simulink model "saturation_mdl"  (R2014a)
settings: Solver=ode45  StartTime=0.0  StopTime=10.0  RelTol=1e-3
values from neighbouring files (symbols this model uses):
  Kg_load_man = 150.5    [simulation.m]
  Kg_noload_man = 245.5    [simulation.m]
libraries: cstblocks x8
settings Model: Creator=daniw  LastModifiedBy=Nino
settings DebuggingCC: UnderspecifiedInitializationDetection=Classic

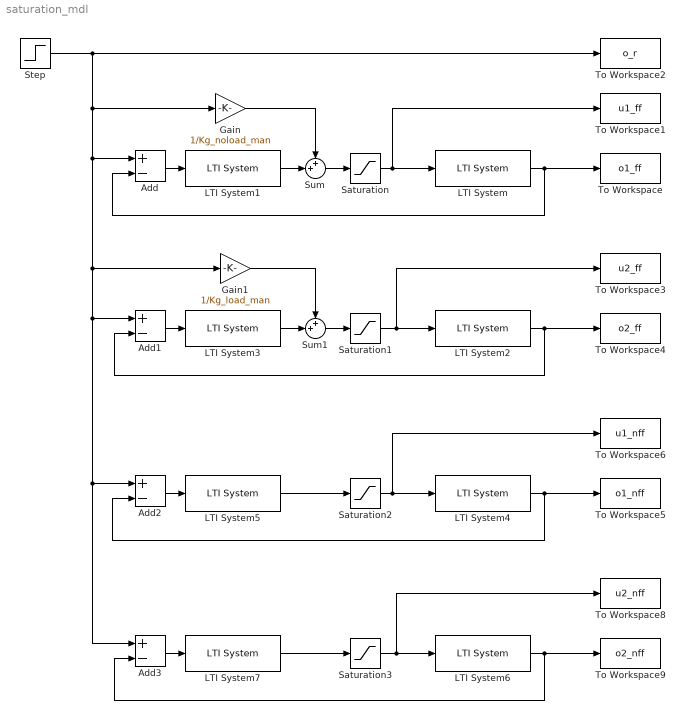
== system saturation_mdl ==
  Add{,1..3} (4 alike) : Sum  Inputs=+-
  Gain : Gain  Gain=1/Kg_noload_man
  Gain1 : Gain  Gain=1/Kg_load_man
  LTI System : cstblocks/LTI System  sys=G11_man  IC=[]
  LTI System{1,3,5,7} (4 alike) : cstblocks/LTI System  sys=C_PI  IC=[]
  LTI System2 : cstblocks/LTI System  sys=G12_man  IC=[]
  LTI System4 : cstblocks/LTI System  sys=G11_man  IC=[]
  LTI System6 : cstblocks/LTI System  sys=G12_man  IC=[]
  Saturation{,1..3} (4 alike) : Saturate  UpperLimit=24  LowerLimit=-24
  Step : Step  After=2500  SampleTime=0
  Sum : Sum  Inputs=++|
  Sum1 : Sum  Inputs=++|
  To Workspace : ToWorkspace  VariableName=o1_ff  SaveFormat=Structure With Time  SampleTime=-1
  To Workspace1 : ToWorkspace  VariableName=u1_ff  SaveFormat=Structure With Time  SampleTime=-1
  To Workspace2 : ToWorkspace  VariableName=o_r  SaveFormat=Structure With Time  SampleTime=-1
  To Workspace3 : ToWorkspace  VariableName=u2_ff  SaveFormat=Structure With Time  SampleTime=-1
  To Workspace4 : ToWorkspace  VariableName=o2_ff  SaveFormat=Structure With Time  SampleTime=-1
  To Workspace5 : ToWorkspace  VariableName=o1_nff  SaveFormat=Structure With Time  SampleTime=-1
  To Workspace6 : ToWorkspace  VariableName=u1_nff  SaveFormat=Structure With Time  SampleTime=-1
  To Workspace8 : ToWorkspace  VariableName=u2_nff  SaveFormat=Structure With Time  SampleTime=-1
  To Workspace9 : ToWorkspace  VariableName=o2_nff  SaveFormat=Structure With Time  SampleTime=-1
  wires:
  Add/1 -> LTI System1/1
  Saturation/1 -> To Workspace1/1, LTI System/1
  LTI System/1 -> To Workspace/1, Add/2
  Add1/1 -> LTI System3/1
  Saturation1/1 -> To Workspace3/1, LTI System2/1
  LTI System2/1 -> To Workspace4/1, Add1/2
  Gain/1 -> Sum/1
  Gain1/1 -> Sum1/1
  LTI System3/1 -> Sum1/2
  Sum1/1 -> Saturation1/1
  LTI System1/1 -> Sum/2
  Sum/1 -> Saturation/1
  Step/1 -> Add/1, Add2/1, Add3/1, Add1/1, Gain1/1, Gain/1, To Workspace2/1
  Add2/1 -> LTI System5/1
  Saturation2/1 -> To Workspace6/1, LTI System4/1
  LTI System4/1 -> To Workspace5/1, Add2/2
  Add3/1 -> LTI System7/1
  Saturation3/1 -> To Workspace8/1, LTI System6/1
  LTI System6/1 -> To Workspace9/1, Add3/2
  LTI System7/1 -> Saturation3/1
  LTI System5/1 -> Saturation2/1
